simulink model "SYSTEM"  (R2026a)
settings: Solver=VariableStepAuto
model workspace (MAT data in the model file):
  CompAir_P : Simulink.ConnectionBus (value not decoded)
  CompAir_S : Simulink.Bus (value not decoded)
  Control_P : Simulink.ConnectionBus (value not decoded)
  Control_S : Simulink.Bus (value not decoded)
  CoolingFW_P : Simulink.ConnectionBus (value not decoded)
  CoolingFW_S : Simulink.Bus (value not decoded)
  FuelOil_P : Simulink.ConnectionBus (value not decoded)
  FuelOil_S : Simulink.Bus (value not decoded)
  Heat_P : Simulink.ConnectionBus (value not decoded)
  Heat_S : Simulink.Bus (value not decoded)
  LubeOil_P : Simulink.ConnectionBus (value not decoded)
  LubeOil_S : Simulink.Bus (value not decoded)
  Physical : Simulink.ConnectionBus (value not decoded)
  Power_P : Simulink.ConnectionBus (value not decoded)
  Power_S : Simulink.Bus (value not decoded)
  SaltWater_P : Simulink.ConnectionBus (value not decoded)
  SaltWater_S : Simulink.Bus (value not decoded)
  WasteGas_P : Simulink.ConnectionBus (value not decoded)
  WasteGas_S : Simulink.Bus (value not decoded)
  WasteOil_P : Simulink.ConnectionBus (value not decoded)
  WasteOil_S : Simulink.Bus (value not decoded)
  WasteSolid_P : Simulink.ConnectionBus (value not decoded)
  WasteSolid_S : Simulink.Bus (value not decoded)
  WasteWater_P : Simulink.ConnectionBus (value not decoded)
  WasteWater_S : Simulink.Bus (value not decoded)
undefined symbols (not defined in the file): FUEL
(part 4 of 5)

== system SYSTEM/SHIP/200 (PROPULSION)/21X (PROPULSORS) ==
  42X-21XC : Inport  OutDataTypeStr=Bus: Control_S
  51X-21XLO : Inport  Port=2  OutDataTypeStr=Bus: LubeOil_S
  53X-21XCA : Inport  Port=3  OutDataTypeStr=Bus: CompAir_S
  50X-21XCFW : Inport  Port=4  OutDataTypeStr=Bus: CoolingFW_S
  21X ABSENT : Subsystem  VariantControl=21X ABSENT
      settings: PortSchema="{\"entries\":[{\"content\":{\"headerSize\":26,\"margin\":15,\"minimumSpacing\":25,\"sides\":[{\"content\":{},\"type\":\"ConnectorPlacement.EquallySpacedRectSide\",\"uuid\":\"c62bca68-e99b-4d4a-8c3b-c9a3c6520291\"},{\"content\":{\"side\":\"RIGHT\"},\"type\":\"ConnectorPlacement.EquallySpacedRectSide\",\"uuid\":\"9f78cd75-5645-4950-8d66-9f0d33627f1f\"},{\"content\":{\"side\":\"TOP\"},\"type\":\"ConnectorPlacement.EquallySpacedRectSide\",\"uuid\":\"f95077c9-4a6b-4bf1-8b13-59697d659817\"},{\"content\":{\"side\":\"BOTTOM\"},\"type\":\"ConnectorPlacement.EquallySpacedRectSide\",\"uuid\":\"6b5f2b68-9ed2-4485-9686-f8a23585a666\"}]},\"type\":\"ConnectorPlacement.EquallySpacedConnector\",\"uuid\":\"da1ef182-4ed3-4fb4-823f-e8eb0a5ecd15\"}],\"packageUris\":[\"http://schema.mathworks.com/mf0/Connector/R2020b\"],\"version\":\"1.0\"}"
  21X ELECTRIC DRIVE : Subsystem  VariantControl=21X ELECTRIC DRIVE
      settings: PortSchema="{\"entries\":[{\"content\":{\"headerSize\":26,\"margin\":15,\"minimumSpacing\":25,\"sides\":[{\"content\":{\"connectorIds\":[\"Out1\"]},\"type\":\"ConnectorPlacement.EquallySpacedRectSide\",\"uuid\":\"c62bca68-e99b-4d4a-8c3b-c9a3c6520291\"},{\"content\":{\"connectorIds\":[\"In1\"],\"side\":\"RIGHT\"},\"type\":\"ConnectorPlacement.EquallySpacedRectSide\",\"uuid\":\"9f78cd75-5645-4950-8d66-9f0d33627f1f\"},{\"content\":{\"connectorIds\":[\"Out4\",\"Out2\",\"Out3\",\"In4\",\"In2\",\"In3\"],\"side\":\"TOP\"},\"type\":\"ConnectorPlacement.EquallySpacedRectSide\",\"uuid\":\"f95077c9-4a6b-4bf1-8b13-59697d659817\"},{\"content\":{\"connectorIds\":[\"RConn1\",\"RConn2\"],\"side\":\"BOTTOM\"},\"type\":\"ConnectorPlacement.EquallySpacedRectSide\",\"uuid\":\"6b5f2b68-9ed2-4485-9686-f8a23585a666\"}]},\"type\":\"ConnectorPlacement.EquallySpacedConnector\",\"uuid\":\"da1ef182-4ed3-4fb4-823f-e8eb0a5ecd15\"}],\"packageUris\":[\"http://schema.mathworks.com/mf0/Connector/R2020b\"],\"version\":\"1.0\"}"
  21X ELECTRIC DRIVE + MANEUVERING THRUSTER : Subsystem  VariantControl=21X ELECTRIC DRIVE + MANUVERING THRUSTER
      settings: PortSchema="{\"entries\":[{\"content\":{\"headerSize\":26,\"margin\":15,\"minimumSpacing\":25,\"sides\":[{\"content\":{\"connectorIds\":[\"Out1\"]},\"type\":\"ConnectorPlacement.EquallySpacedRectSide\",\"uuid\":\"c62bca68-e99b-4d4a-8c3b-c9a3c6520291\"},{\"content\":{\"connectorIds\":[\"In1\"],\"side\":\"RIGHT\"},\"type\":\"ConnectorPlacement.EquallySpacedRectSide\",\"uuid\":\"9f78cd75-5645-4950-8d66-9f0d33627f1f\"},{\"content\":{\"connectorIds\":[\"Out4\",\"Out2\",\"Out3\",\"In4\",\"In2\",\"In3\"],\"side\":\"TOP\"},\"type\":\"ConnectorPlacement.EquallySpacedRectSide\",\"uuid\":\"f95077c9-4a6b-4bf1-8b13-59697d659817\"},{\"content\":{\"connectorIds\":[\"RConn1\",\"RConn2\"],\"side\":\"BOTTOM\"},\"type\":\"ConnectorPlacement.EquallySpacedRectSide\",\"uuid\":\"6b5f2b68-9ed2-4485-9686-f8a23585a666\"}]},\"type\":\"ConnectorPlacement.EquallySpacedConnector\",\"uuid\":\"da1ef182-4ed3-4fb4-823f-e8eb0a5ecd15\"}],\"packageUris\":[\"http://schema.mathworks.com/mf0/Connector/R2020b\"],\"version\":\"1.0\"}"
  21X SHAFT DRIVE : Subsystem  VariantControl=21X SHAFT DRIVE
      settings: PortSchema="{\"entries\":[{\"content\":{\"headerSize\":26,\"margin\":15,\"minimumSpacing\":25,\"sides\":[{\"content\":{\"connectorIds\":[\"Out1\"]},\"type\":\"ConnectorPlacement.EquallySpacedRectSide\",\"uuid\":\"c62bca68-e99b-4d4a-8c3b-c9a3c6520291\"},{\"content\":{\"connectorIds\":[\"In1\"],\"side\":\"RIGHT\"},\"type\":\"ConnectorPlacement.EquallySpacedRectSide\",\"uuid\":\"9f78cd75-5645-4950-8d66-9f0d33627f1f\"},{\"content\":{\"connectorIds\":[\"Out4\",\"Out2\",\"Out3\",\"In4\",\"In2\",\"In3\"],\"side\":\"TOP\"},\"type\":\"ConnectorPlacement.EquallySpacedRectSide\",\"uuid\":\"f95077c9-4a6b-4bf1-8b13-59697d659817\"},{\"content\":{\"connectorIds\":[\"RConn1\",\"RConn2\"],\"side\":\"BOTTOM\"},\"type\":\"ConnectorPlacement.EquallySpacedRectSide\",\"uuid\":\"6b5f2b68-9ed2-4485-9686-f8a23585a666\"}]},\"type\":\"ConnectorPlacement.EquallySpacedConnector\",\"uuid\":\"da1ef182-4ed3-4fb4-823f-e8eb0a5ecd15\"}],\"packageUris\":[\"http://schema.mathworks.com/mf0/Connector/R2020b\"],\"version\":\"1.0\"}"
  21X SHAFT DRIVE + MANEUVERING THRUSTER : Subsystem  VariantControl=21X SHAFT DRIVE + MANUVERING THRUSTER
      settings: PortSchema="{\"entries\":[{\"content\":{\"headerSize\":26,\"margin\":15,\"minimumSpacing\":25,\"sides\":[{\"content\":{\"connectorIds\":[\"Out1\"]},\"type\":\"ConnectorPlacement.EquallySpacedRectSide\",\"uuid\":\"c62bca68-e99b-4d4a-8c3b-c9a3c6520291\"},{\"content\":{\"connectorIds\":[\"In1\"],\"side\":\"RIGHT\"},\"type\":\"ConnectorPlacement.EquallySpacedRectSide\",\"uuid\":\"9f78cd75-5645-4950-8d66-9f0d33627f1f\"},{\"content\":{\"connectorIds\":[\"Out4\",\"Out2\",\"Out3\",\"In4\",\"In2\",\"In3\"],\"side\":\"TOP\"},\"type\":\"ConnectorPlacement.EquallySpacedRectSide\",\"uuid\":\"f95077c9-4a6b-4bf1-8b13-59697d659817\"},{\"content\":{\"connectorIds\":[\"RConn1\",\"RConn2\"],\"side\":\"BOTTOM\"},\"type\":\"ConnectorPlacement.EquallySpacedRectSide\",\"uuid\":\"6b5f2b68-9ed2-4485-9686-f8a23585a666\"}]},\"type\":\"ConnectorPlacement.EquallySpacedConnector\",\"uuid\":\"da1ef182-4ed3-4fb4-823f-e8eb0a5ecd15\"}],\"packageUris\":[\"http://schema.mathworks.com/mf0/Connector/R2020b\"],\"version\":\"1.0\"}"
  21X WATER JET : Subsystem  VariantControl=21X WATER JET
      settings: PortSchema="{\"entries\":[{\"content\":{\"headerSize\":26,\"margin\":15,\"minimumSpacing\":25,\"sides\":[{\"content\":{\"connectorIds\":[\"Out1\"]},\"type\":\"ConnectorPlacement.EquallySpacedRectSide\",\"uuid\":\"c62bca68-e99b-4d4a-8c3b-c9a3c6520291\"},{\"content\":{\"connectorIds\":[\"In1\"],\"side\":\"RIGHT\"},\"type\":\"ConnectorPlacement.EquallySpacedRectSide\",\"uuid\":\"9f78cd75-5645-4950-8d66-9f0d33627f1f\"},{\"content\":{\"connectorIds\":[\"Out4\",\"Out2\",\"Out3\",\"In4\",\"In2\",\"In3\"],\"side\":\"TOP\"},\"type\":\"ConnectorPlacement.EquallySpacedRectSide\",\"uuid\":\"f95077c9-4a6b-4bf1-8b13-59697d659817\"},{\"content\":{\"connectorIds\":[\"RConn1\",\"RConn2\"],\"side\":\"BOTTOM\"},\"type\":\"ConnectorPlacement.EquallySpacedRectSide\",\"uuid\":\"6b5f2b68-9ed2-4485-9686-f8a23585a666\"}]},\"type\":\"ConnectorPlacement.EquallySpacedConnector\",\"uuid\":\"da1ef182-4ed3-4fb4-823f-e8eb0a5ecd15\"}],\"packageUris\":[\"http://schema.mathworks.com/mf0/Connector/R2020b\"],\"version\":\"1.0\"}"
  21X WATER JET + MANEUVERING THRUSTER : Subsystem  VariantControl=21X WATER JET + MANUVERING THRUSTER
      settings: PortSchema="{\"entries\":[{\"content\":{\"headerSize\":26,\"margin\":15,\"minimumSpacing\":25,\"sides\":[{\"content\":{\"connectorIds\":[\"Out1\"]},\"type\":\"ConnectorPlacement.EquallySpacedRectSide\",\"uuid\":\"c62bca68-e99b-4d4a-8c3b-c9a3c6520291\"},{\"content\":{\"connectorIds\":[\"In1\"],\"side\":\"RIGHT\"},\"type\":\"ConnectorPlacement.EquallySpacedRectSide\",\"uuid\":\"9f78cd75-5645-4950-8d66-9f0d33627f1f\"},{\"content\":{\"connectorIds\":[\"Out4\",\"Out2\",\"Out3\",\"In4\",\"In2\",\"In3\"],\"side\":\"TOP\"},\"type\":\"ConnectorPlacement.EquallySpacedRectSide\",\"uuid\":\"f95077c9-4a6b-4bf1-8b13-59697d659817\"},{\"content\":{\"connectorIds\":[\"RConn1\",\"RConn2\"],\"side\":\"BOTTOM\"},\"type\":\"ConnectorPlacement.EquallySpacedRectSide\",\"uuid\":\"6b5f2b68-9ed2-4485-9686-f8a23585a666\"}]},\"type\":\"ConnectorPlacement.EquallySpacedConnector\",\"uuid\":\"da1ef182-4ed3-4fb4-823f-e8eb0a5ecd15\"}],\"packageUris\":[\"http://schema.mathworks.com/mf0/Connector/R2020b\"],\"version\":\"1.0\"}"
  10X-21X : PMIOPort  Side=Right  ConnectionType=Bus: Physical
  FROM 22X : PMIOPort  Port=2  Side=Right  ConnectionType=Bus: Physical
  21X-42XC : Outport  OutDataTypeStr=Bus: Control_S
  21X-51XLO : Outport  Port=2  OutDataTypeStr=Bus: LubeOil_S
  21X-53XCA : Outport  Port=3  OutDataTypeStr=Bus: CompAir_S
  21X-50XCFW : Outport  Port=4  OutDataTypeStr=Bus: CoolingFW_S

== system SYSTEM/SHIP/200 (PROPULSION)/22X (SHAFTING) ==
  51X-22XLO : Inport  OutDataTypeStr=Bus: LubeOil_S
  53X-22XCA : Inport  Port=2  OutDataTypeStr=Bus: CompAir_S
  22X ABSENT : Subsystem  VariantControl=22X ABSENT
      settings: PortSchema="{\"entries\":[{\"content\":{\"headerSize\":26,\"margin\":15,\"minimumSpacing\":25,\"sides\":[{\"content\":{},\"type\":\"ConnectorPlacement.EquallySpacedRectSide\",\"uuid\":\"c62bca68-e99b-4d4a-8c3b-c9a3c6520291\"},{\"content\":{\"side\":\"RIGHT\"},\"type\":\"ConnectorPlacement.EquallySpacedRectSide\",\"uuid\":\"9f78cd75-5645-4950-8d66-9f0d33627f1f\"},{\"content\":{\"side\":\"TOP\"},\"type\":\"ConnectorPlacement.EquallySpacedRectSide\",\"uuid\":\"f95077c9-4a6b-4bf1-8b13-59697d659817\"},{\"content\":{\"side\":\"BOTTOM\"},\"type\":\"ConnectorPlacement.EquallySpacedRectSide\",\"uuid\":\"1f93f758-4269-498d-aa3c-a1654d57bbcc\"}]},\"type\":\"ConnectorPlacement.EquallySpacedConnector\",\"uuid\":\"da1ef182-4ed3-4fb4-823f-e8eb0a5ecd15\"}],\"packageUris\":[\"http://schema.mathworks.com/mf0/Connector/R2020b\"],\"version\":\"1.0\"}"
  22X MECHANICAL : Subsystem  VariantControl=22X MECHANICAL
      settings: PortSchema="{\"entries\":[{\"content\":{\"headerSize\":26,\"margin\":15,\"minimumSpacing\":25,\"sides\":[{\"content\":{\"connectorIds\":[\"Out3\"]},\"type\":\"ConnectorPlacement.EquallySpacedRectSide\",\"uuid\":\"c62bca68-e99b-4d4a-8c3b-c9a3c6520291\"},{\"content\":{\"side\":\"RIGHT\"},\"type\":\"ConnectorPlacement.EquallySpacedRectSide\",\"uuid\":\"9f78cd75-5645-4950-8d66-9f0d33627f1f\"},{\"content\":{\"connectorIds\":[\"Out1\",\"Out2\",\"In1\",\"In2\"],\"side\":\"TOP\"},\"type\":\"ConnectorPlacement.EquallySpacedRectSide\",\"uuid\":\"f95077c9-4a6b-4bf1-8b13-59697d659817\"},{\"content\":{\"connectorIds\":[\"RConn3\",\"RConn2\",\"RConn1\"],\"side\":\"BOTTOM\"},\"type\":\"ConnectorPlacement.EquallySpacedRectSide\",\"uuid\":\"1f93f758-4269-498d-aa3c-a1654d57bbcc\"}]},\"type\":\"ConnectorPlacement.EquallySpacedConnector\",\"uuid\":\"da1ef182-4ed3-4fb4-823f-e8eb0a5ecd15\"}],\"packageUris\":[\"http://schema.mathworks.com/mf0/Connector/R2020b\"],\"version\":\"1.0\"}"
  TOFROM 23X : PMIOPort  Side=Right  ConnectionType=Bus: Physical
  10X-22X : PMIOPort  Port=2  Side=Right  ConnectionType=Bus: Physical
  TO 21X : PMIOPort  Port=3  Side=Right  ConnectionType=Bus: Physical
  22X-51XLO : Outport  OutDataTypeStr=Bus: LubeOil_S
  22X-53XCA : Outport  Port=2  OutDataTypeStr=Bus: CompAir_S
  22X-42XC : Outport  Port=3  OutDataTypeStr=Bus: Control_S

== system SYSTEM/SHIP/200 (PROPULSION)/23X (POWER TRANSMISSION) ==
  51X-23XLO : Inport  OutDataTypeStr=Bus: LubeOil_S
  42X-23XC : Inport  Port=2  OutDataTypeStr=Bus: Control_S
  23X ABSENT : Subsystem  VariantControl=23X ABSENT
      settings: PortSchema="{\"entries\":[{\"content\":{\"headerSize\":26,\"margin\":15,\"minimumSpacing\":25,\"sides\":[{\"content\":{},\"type\":\"ConnectorPlacement.EquallySpacedRectSide\",\"uuid\":\"c62bca68-e99b-4d4a-8c3b-c9a3c6520291\"},{\"content\":{\"side\":\"RIGHT\"},\"type\":\"ConnectorPlacement.EquallySpacedRectSide\",\"uuid\":\"9f78cd75-5645-4950-8d66-9f0d33627f1f\"},{\"content\":{\"side\":\"TOP\"},\"type\":\"ConnectorPlacement.EquallySpacedRectSide\",\"uuid\":\"f95077c9-4a6b-4bf1-8b13-59697d659817\"},{\"content\":{\"side\":\"BOTTOM\"},\"type\":\"ConnectorPlacement.EquallySpacedRectSide\",\"uuid\":\"886e986c-d088-4ccd-a11a-30cba32770e8\"}]},\"type\":\"ConnectorPlacement.EquallySpacedConnector\",\"uuid\":\"da1ef182-4ed3-4fb4-823f-e8eb0a5ecd15\"}],\"packageUris\":[\"http://schema.mathworks.com/mf0/Connector/R2020b\"],\"version\":\"1.0\"}"
  23X MECHANICAL : Subsystem  VariantControl=23X MECHANICAL
      settings: PortSchema="{\"entries\":[{\"content\":{\"headerSize\":26,\"margin\":15,\"minimumSpacing\":25,\"sides\":[{\"content\":{\"connectorIds\":[\"Out2\"]},\"type\":\"ConnectorPlacement.EquallySpacedRectSide\",\"uuid\":\"c62bca68-e99b-4d4a-8c3b-c9a3c6520291\"},{\"content\":{\"connectorIds\":[\"Out3\",\"In2\"],\"side\":\"RIGHT\"},\"type\":\"ConnectorPlacement.EquallySpacedRectSide\",\"uuid\":\"9f78cd75-5645-4950-8d66-9f0d33627f1f\"},{\"content\":{\"connectorIds\":[\"Out1\",\"In1\"],\"side\":\"TOP\"},\"type\":\"ConnectorPlacement.EquallySpacedRectSide\",\"uuid\":\"f95077c9-4a6b-4bf1-8b13-59697d659817\"},{\"content\":{\"connectorIds\":[\"LConn2\",\"LConn1\",\"RConn1\"],\"side\":\"BOTTOM\"},\"type\":\"ConnectorPlacement.EquallySpacedRectSide\",\"uuid\":\"886e986c-d088-4ccd-a11a-30cba32770e8\"}]},\"type\":\"ConnectorPlacement.EquallySpacedConnector\",\"uuid\":\"da1ef182-4ed3-4fb4-823f-e8eb0a5ecd15\"}],\"packageUris\":[\"http://schema.mathworks.com/mf0/Connector/R2020b\"],\"version\":\"1.0\"}"
  23X MECHANICAL WITH POWER TAKEOFF : Subsystem  VariantControl=23X MECHANICAL WITH POWER TAKEOFF
      settings: PortSchema="{\"entries\":[{\"content\":{\"headerSize\":26,\"margin\":15,\"minimumSpacing\":25,\"sides\":[{\"content\":{\"connectorIds\":[\"Out2\"]},\"type\":\"ConnectorPlacement.EquallySpacedRectSide\",\"uuid\":\"c62bca68-e99b-4d4a-8c3b-c9a3c6520291\"},{\"content\":{\"connectorIds\":[\"Out3\",\"In2\"],\"side\":\"RIGHT\"},\"type\":\"ConnectorPlacement.EquallySpacedRectSide\",\"uuid\":\"9f78cd75-5645-4950-8d66-9f0d33627f1f\"},{\"content\":{\"connectorIds\":[\"Out1\",\"In1\"],\"side\":\"TOP\"},\"type\":\"ConnectorPlacement.EquallySpacedRectSide\",\"uuid\":\"f95077c9-4a6b-4bf1-8b13-59697d659817\"},{\"content\":{\"connectorIds\":[\"LConn2\",\"LConn1\",\"RConn1\"],\"side\":\"BOTTOM\"},\"type\":\"ConnectorPlacement.EquallySpacedRectSide\",\"uuid\":\"886e986c-d088-4ccd-a11a-30cba32770e8\"}]},\"type\":\"ConnectorPlacement.EquallySpacedConnector\",\"uuid\":\"da1ef182-4ed3-4fb4-823f-e8eb0a5ecd15\"}],\"packageUris\":[\"http://schema.mathworks.com/mf0/Connector/R2020b\"],\"version\":\"1.0\"}"
  TOFROM 22X : PMIOPort  Side=Left  ConnectionType=Bus: Physical
  FROM 20X : PMIOPort  Port=2  Side=Left  ConnectionType=Bus: Physical
  10X-23X : PMIOPort  Port=3  Side=Right  ConnectionType=Bus: Physical
  23X-51XLO : Outport  OutDataTypeStr=Bus: LubeOil_S
  23X-42XC : Outport  Port=2  OutDataTypeStr=Bus: Control_S
  23X-31XP : Outport  Port=3  OutDataTypeStr=Bus: Power_S

== system SYSTEM/SHIP/300 (ELECTRICAL)/30X (GENERATOR SETS) ==
  Bus Element In1 : Inport  PortName=42X-30XC
  Bus Element In3 : Inport  Port=2  PortName=51X-30XLO
  Bus Element In5 : Inport  Port=3  PortName=53X-30XCA
  Bus Element In4 : Inport  Port=4  PortName=52X-30XFO
  Bus Element In2 : Inport  Port=5  PortName=50X-30XCFW
  10X-30X : PMIOPort  Side=Right  ConnectionType=Bus: Physical
  30X-526FO : PMIOPort  Port=2  Side=Left  ConnectionType=Bus: FuelOil_P
  526-30XFO : PMIOPort  Port=3  Side=Left  ConnectionType=Bus: FuelOil_P
  Bus Element Out2 : Outport  PortName=30X-42XC
  Bus Element Out4 : Outport  Port=2  PortName=30X-51XLO
  Bus Element Out5 : Outport  Port=3  PortName=30X-52XFO
  Bus Element Out6 : Outport  Port=4  PortName=30X-53XCA
  Bus Element Out7 : Outport  Port=5  PortName=30X-57XWG
  Bus Element Out3 : Outport  Port=6  PortName=30X-50XCFW
  Bus Element Out1 : Outport  Port=7  PortName=30X-31XP

== system SYSTEM/SHIP/300 (ELECTRICAL)/31X (POWER DISTRIBUTION) ==
  Bus Element In3 : Inport  PortName=23X-31XP
  Bus Element In4 : Inport  Port=2  PortName=32X-31XP
  Bus Element In5 : Inport  Port=3  PortName=42X-31XC
  Bus Element In1 : Inport  Port=4  PortName=30X-31XP
  Bus Element In2 : Inport  Port=5  PortName=33X-31XP
  10X-31X : PMIOPort  Side=Right  ConnectionType=Bus: Physical
  Bus Element Out25 : Outport  PortName=31X-42XC
  Bus Element Out3 : Outport  Port=2  PortName=31X-40XP
  Bus Element Out4 : Outport  Port=3  PortName=31X-41XP
  Bus Element Out5 : Outport  Port=4  PortName=31X-42XP
  Bus Element Out6 : Outport  Port=5  PortName=31X-43XP
  Bus Element Out7 : Outport  Port=6  PortName=31X-44XP
  Bus Element Out2 : Outport  Port=7  PortName=31X-45XP
  Bus Element Out8 : Outport  Port=8  PortName=31X-50XP
  Bus Element Out9 : Outport  Port=9  PortName=31X-51XP
  Bus Element Out10 : Outport  Port=10  PortName=31X-529P
  Bus Element Out11 : Outport  Port=11  PortName=31X-53XP
  Bus Element Out12 : Outport  Port=12  PortName=31X-54XP
  Bus Element Out13 : Outport  Port=13  PortName=31X-55XP
  Bus Element Out14 : Outport  Port=14  PortName=31X-56XP
  Bus Element Out15 : Outport  Port=15  PortName=31X-57XP
  Bus Element Out16 : Outport  Port=16  PortName=31X-58XP
  Bus Element Out17 : Outport  Port=17  PortName=31X-59XP
  Bus Element Out18 : Outport  Port=18  PortName=31X-60XP
  Bus Element Out19 : Outport  Port=19  PortName=31X-61XP
  Bus Element Out20 : Outport  Port=20  PortName=31X-70XP
  Bus Element Out21 : Outport  Port=21  PortName=31X-71XP
  Bus Element Out22 : Outport  Port=22  PortName=31X-72XP
  Bus Element Out23 : Outport  Port=23  PortName=31X-73XP
  Bus Element Out24 : Outport  Port=24  PortName=31X-74XP
  Bus Element Out1 : Outport  Port=25  PortName=31X-32XP

== system SYSTEM/SHIP/300 (ELECTRICAL)/32X (BATTERY) ==
  Bus Element In2 : Inport  PortName=42X-32XC
  Bus Element In1 : Inport  Port=2  PortName=31X-32XP
  10X-32X : PMIOPort  Side=Right  ConnectionType=Bus: Physical
  Bus Element Out1 : Outport  PortName=32X-31XP
  Bus Element Out2 : Outport  Port=2  PortName=32X-42XC

== system SYSTEM/SHIP/300 (ELECTRICAL)/33X (SHORE POWER) ==
  Bus Element In1 : Inport  PortName=42X-33XC
  10X-33X : PMIOPort  Side=Right  ConnectionType=Bus: Physical
  Bus Element Out2 : Outport  PortName=33X-42XC
  Bus Element Out1 : Outport  Port=2  PortName=33X-31XP

== system SYSTEM/SHIP/400 (COMMAND CONTROL)/40X (NAVIGATION//AIS) ==
  Bus Element In3 : Inport  PortName=53X-40XCA
  Bus Element In2 : Inport  Port=2  PortName=42X-40XC
  Bus Element In1 : Inport  Port=3  PortName=31X-40XP
  10X-40X : PMIOPort  Side=Right  ConnectionType=Bus: Physical
  Bus Element Out2 : Outport  PortName=40X-53XCA
  Bus Element Out1 : Outport  Port=2  PortName=40X-42XC

== system SYSTEM/SHIP/400 (COMMAND CONTROL)/41X (RADIO//SATCOM) ==
  Bus Element In2 : Inport  PortName=42X-41XC
  Bus Element In1 : Inport  Port=2  PortName=31X-41XP
  10X-41X : PMIOPort  Side=Right  ConnectionType=Bus: Physical
  Bus Element Out1 : Outport  PortName=41X-42XC

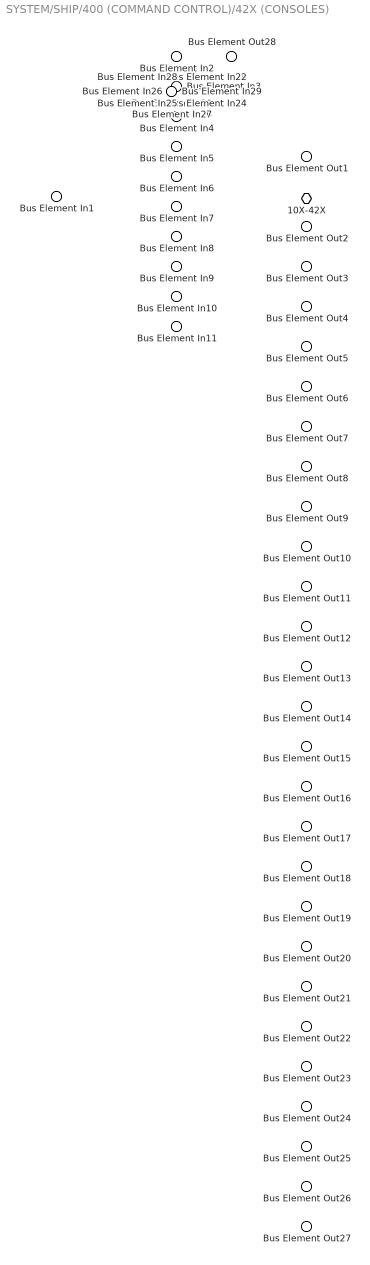
== system SYSTEM/SHIP/400 (COMMAND CONTROL)/42X (CONSOLES) ==
  Bus Element In30 : Inport  PortName=50X-42XCFW
  Bus Element In2 : Inport  Port=2  PortName=41X-42XC
  Bus Element In3 : Inport  Port=3  PortName=40X-42XC
  Bus Element In4 : Inport  Port=4  PortName=43X-42XC
  Bus Element In5 : Inport  Port=5  PortName=44X-42XC
  Bus Element In6 : Inport  Port=6  PortName=45X-42XC
  Bus Element In7 : Inport  Port=7  PortName=20X-42XC
  Bus Element In8 : Inport  Port=8  PortName=21X-42XC
  Bus Element In10 : Inport  Port=9  PortName=22X-42XC
  Bus Element In9 : Inport  Port=10  PortName=23X-42XC
  Bus Element In11 : Inport  Port=11  PortName=30X-42XC
  Bus Element In12 : Inport  Port=12  PortName=31X-42XC
  Bus Element In13 : Inport  Port=13  PortName=32X-42XC
  Bus Element In14 : Inport  Port=14  PortName=33X-42XC
  Bus Element In15 : Inport  Port=15  PortName=50X-42XC
  Bus Element In16 : Inport  Port=16  PortName=51X-42XC
  Bus Element In17 : Inport  Port=17  PortName=528-42XC
  Bus Element In18 : Inport  Port=18  PortName=53X-42XC
  Bus Element In19 : Inport  Port=19  PortName=54X-42XC
  Bus Element In20 : Inport  Port=20  PortName=55X-42XC
  Bus Element In21 : Inport  Port=21  PortName=56X-42XC
  Bus Element In22 : Inport  Port=22  PortName=57X-42XC
  Bus Element In23 : Inport  Port=23  PortName=58X-42XC
  Bus Element In24 : Inport  Port=24  PortName=59X-42XC
  Bus Element In25 : Inport  Port=25  PortName=70X-42XC
  Bus Element In26 : Inport  Port=26  PortName=71X-42XC
  Bus Element In27 : Inport  Port=27  PortName=72X-42XC
  Bus Element In28 : Inport  Port=28  PortName=73X-42XC
  Bus Element In29 : Inport  Port=29  PortName=74X-42XC
  Bus Element In1 : Inport  Port=30  PortName=31X-42XP
  10X-42X : PMIOPort  Side=Right  ConnectionType=Bus: Physical
  Bus Element Out28 : Outport  PortName=42X-50XCFW
  Bus Element Out1 : Outport  Port=2  PortName=42X-40XC
  Bus Element Out2 : Outport  Port=3  PortName=42X-41XC
  Bus Element Out3 : Outport  Port=4  PortName=42X-43XC
  Bus Element Out4 : Outport  Port=5  PortName=42X-44XC
  Bus Element Out5 : Outport  Port=6  PortName=42X-45XC
  Bus Element Out6 : Outport  Port=7  PortName=42X-20XC
  Bus Element Out7 : Outport  Port=8  PortName=42X-21XC
  Bus Element Out8 : Outport  Port=9  PortName=42X-23XC
  Bus Element Out9 : Outport  Port=10  PortName=42X-30XC
  Bus Element Out10 : Outport  Port=11  PortName=42X-31XC
  Bus Element Out11 : Outport  Port=12  PortName=42X-32XC
  Bus Element Out12 : Outport  Port=13  PortName=42X-33XC
  Bus Element Out13 : Outport  Port=14  PortName=42X-50XC
  Bus Element Out14 : Outport  Port=15  PortName=42X-51XC
  Bus Element Out15 : Outport  Port=16  PortName=42X-528C
  Bus Element Out16 : Outport  Port=17  PortName=42X-53XC
  Bus Element Out17 : Outport  Port=18  PortName=42X-54XC
  Bus Element Out18 : Outport  Port=19  PortName=42X-55XC
  Bus Element Out19 : Outport  Port=20  PortName=42X-56XC
  Bus Element Out20 : Outport  Port=21  PortName=42X-57XC
  Bus Element Out21 : Outport  Port=22  PortName=42X-58XC
  Bus Element Out22 : Outport  Port=23  PortName=42X-59XC
  Bus Element Out23 : Outport  Port=24  PortName=42X-70XC
  Bus Element Out24 : Outport  Port=25  PortName=42X-71XC
  Bus Element Out25 : Outport  Port=26  PortName=42X-72XC
  Bus Element Out26 : Outport  Port=27  PortName=42X-73XC
  Bus Element Out27 : Outport  Port=28  PortName=42X-74XC

== system SYSTEM/SHIP/400 (COMMAND CONTROL)/43X (STEERAGE) ==
  Bus Element In2 : Inport  PortName=42X-43XC
  Bus Element In4 : Inport  Port=2  PortName=51X-43XLO
  Bus Element In3 : Inport  Port=3  PortName=50X-43XCFW
  Bus Element In1 : Inport  Port=4  PortName=31X-43XP
  10X-43X : PMIOPort  Side=Right  ConnectionType=Bus: Physical
  Bus Element Out1 : Outport  PortName=43X-42XC
  Bus Element Out3 : Outport  Port=2  PortName=43X-51XLO
  Bus Element Out2 : Outport  Port=3  PortName=43X-50XCFW

== system SYSTEM/SHIP/400 (COMMAND CONTROL)/44X (AIR SURVEILLANCE) ==
  Bus Element In3 : Inport  PortName=50X-44XCFW
  Bus Element In2 : Inport  Port=2  PortName=42X-44XC
  Bus Element In1 : Inport  Port=3  PortName=31X-44XP
  10X-44X : PMIOPort  Side=Right  ConnectionType=Bus: Physical
  Bus Element Out2 : Outport  PortName=44X-50XCFW
  Bus Element Out1 : Outport  Port=2  PortName=44X-42XC

== system SYSTEM/SHIP/400 (COMMAND CONTROL)/45X (WATER SURVEILLANCE) ==
  Bus Element In2 : Inport  PortName=42X-45XC
  Bus Element In1 : Inport  Port=2  PortName=31X-45XP
  10X-45X : PMIOPort  Side=Right  ConnectionType=Bus: Physical
  Bus Element Out1 : Outport  PortName=45X-42XC

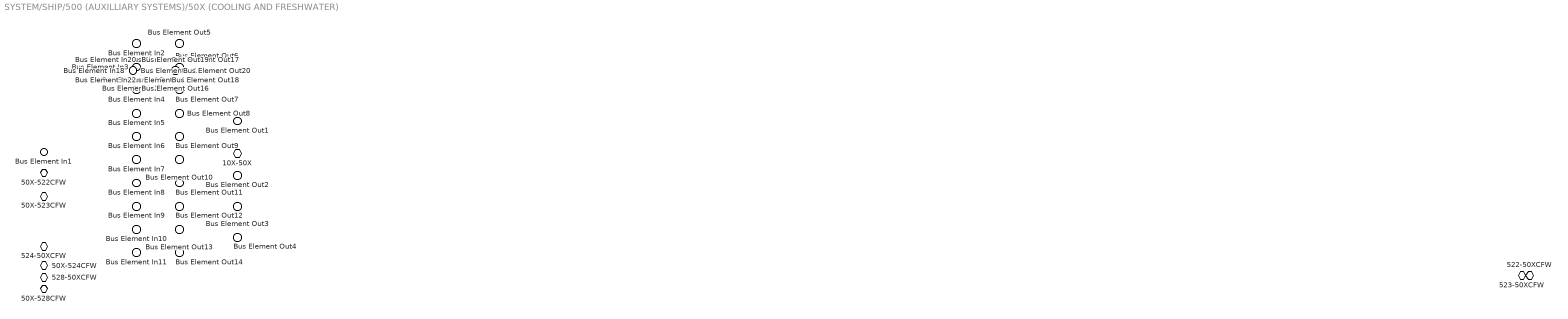
== system SYSTEM/SHIP/500 (AUXILLIARY SYSTEMS)/50X (COOLING AND FRESHWATER) ==
  Bus Element In2 : Inport  PortName=42X-50XC
  Bus Element In3 : Inport  Port=2  PortName=20X-50XCFW
  Bus Element In4 : Inport  Port=3  PortName=21X-50XCFW
  Bus Element In16 : Inport  Port=4  PortName=42X-50XCFW
  Bus Element In6 : Inport  Port=5  PortName=43X-50XCFW
  Bus Element In17 : Inport  Port=6  PortName=44X-50XCFW
  Bus Element In7 : Inport  Port=7  PortName=51X-50XCFW
  Bus Element In23 : Inport  Port=8  PortName=51X-50XLO
  Bus Element In8 : Inport  Port=9  PortName=52X-50XCFW
  Bus Element In9 : Inport  Port=10  PortName=53X-50XCFW
  Bus Element In10 : Inport  Port=11  PortName=54X-50XSW
  Bus Element In11 : Inport  Port=12  PortName=54X-50XCFW
  Bus Element In12 : Inport  Port=13  PortName=55X-50XCFW
  Bus Element In13 : Inport  Port=14  PortName=57X-50XCFW
  Bus Element In14 : Inport  Port=15  PortName=58X-50XCFW
  Bus Element In15 : Inport  Port=16  PortName=59X-50XCFW
  Bus Element In22 : Inport  Port=17  PortName=60X-50XCFW
  Bus Element In21 : Inport  Port=18  PortName=61X-50XCFW
  Bus Element In20 : Inport  Port=19  PortName=71X-50XCFW
  Bus Element In19 : Inport  Port=20  PortName=72X-50XCFW
  Bus Element In18 : Inport  Port=21  PortName=73X-50XCFW
  Bus Element In5 : Inport  Port=22  PortName=30X-50XCFW
  Bus Element In1 : Inport  Port=23  PortName=31X-50XP
  10X-50X : PMIOPort  Side=Right  ConnectionType=Bus: Physical
  50X-522CFW : PMIOPort  Port=2  Side=Left  ConnectionType=Bus: CoolingFW_P
  50X-523CFW : PMIOPort  Port=3  Side=Left  ConnectionType=Bus: CoolingFW_P
  50X-524CFW : PMIOPort  Port=4  Side=Left  ConnectionType=Bus: CoolingFW_P
  50X-528CFW : PMIOPort  Port=5  Side=Left  ConnectionType=Bus: CoolingFW_P
  522-50XCFW : PMIOPort  Port=6  Side=Left  ConnectionType=Bus: CoolingFW_P
  523-50XCFW : PMIOPort  Port=7  Side=Left  ConnectionType=Bus: CoolingFW_P
  524-50XCFW : PMIOPort  Port=8  Side=Left  ConnectionType=Bus: CoolingFW_P
  528-50XCFW : PMIOPort  Port=9  Side=Left  ConnectionType=Bus: CoolingFW_P
  Bus Element Out1 : Outport  PortName=50X-42XC
  Bus Element Out2 : Outport  Port=2  PortName=50X-20XCFW
  Bus Element Out3 : Outport  Port=3  PortName=50X-21XCFW
  Bus Element Out14 : Outport  Port=4  PortName=50X-42XCFW
  Bus Element Out5 : Outport  Port=5  PortName=50X-43XCFW
  Bus Element Out15 : Outport  Port=6  PortName=50X-44XCFW
  Bus Element Out6 : Outport  Port=7  PortName=50X-51XCFW
  Bus Element Out21 : Outport  Port=8  PortName=50X-51XLO
  Bus Element Out7 : Outport  Port=9  PortName=50X-52XCFW
  Bus Element Out8 : Outport  Port=10  PortName=50X-53XCFW
  Bus Element Out9 : Outport  Port=11  PortName=50X-54XCFW
  Bus Element Out10 : Outport  Port=12  PortName=50X-55XCFW
  Bus Element Out11 : Outport  Port=13  PortName=50X-57XCFW
  Bus Element Out12 : Outport  Port=14  PortName=50X-58XCFW
  Bus Element Out13 : Outport  Port=15  PortName=50X-59XCFW
  Bus Element Out16 : Outport  Port=16  PortName=50X-60XCFW
  Bus Element Out17 : Outport  Port=17  PortName=50X-61XCFW
  Bus Element Out18 : Outport  Port=18  PortName=50X-71XCFW
  Bus Element Out19 : Outport  Port=19  PortName=50X-72XCFW
  Bus Element Out20 : Outport  Port=20  PortName=50X-73XCFW
  Bus Element Out4 : Outport  Port=21  PortName=50X-30XCFW

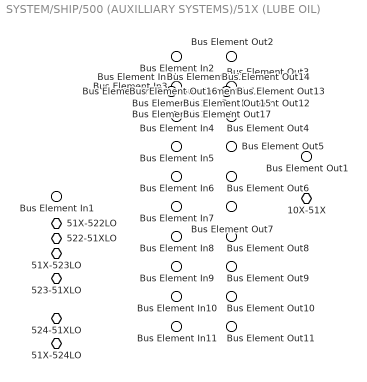
== system SYSTEM/SHIP/500 (AUXILLIARY SYSTEMS)/51X (LUBE OIL) ==
  Bus Element In4 : Inport  PortName=20X-51XLO
  Bus Element In5 : Inport  Port=2  PortName=21X-51XLO
  Bus Element In6 : Inport  Port=3  PortName=22X-51XLO
  Bus Element In7 : Inport  Port=4  PortName=23X-51XLO
  Bus Element In8 : Inport  Port=5  PortName=30X-51XLO
  Bus Element In9 : Inport  Port=6  PortName=43X-51XLO
  Bus Element In3 : Inport  Port=7  PortName=50X-51XCFW
  Bus Element In10 : Inport  Port=8  PortName=50X-51XLO
  Bus Element In11 : Inport  Port=9  PortName=52X-51XLO
  Bus Element In12 : Inport  Port=10  PortName=53X-51XLO
  Bus Element In13 : Inport  Port=11  PortName=54X-51XLO
  Bus Element In14 : Inport  Port=12  PortName=55X-51XLO
  Bus Element In15 : Inport  Port=13  PortName=57X-51XLO
  Bus Element In16 : Inport  Port=14  PortName=58X-51XLO
  Bus Element In17 : Inport  Port=15  PortName=59X-51XLO
  Bus Element In2 : Inport  Port=16  PortName=42X-51XC
  Bus Element In1 : Inport  Port=17  PortName=31X-51XP
  10X-51X : PMIOPort  Side=Right  ConnectionType=Bus: Physical
  51X-522LO : PMIOPort  Port=2  Side=Left  ConnectionType=Bus: LubeOil_P
  51X-523LO : PMIOPort  Port=3  Side=Left  ConnectionType=Bus: LubeOil_P
  51X-524LO : PMIOPort  Port=4  Side=Left  ConnectionType=Bus: LubeOil_P
  522-51XLO : PMIOPort  Port=5  Side=Left  ConnectionType=Bus: LubeOil_P
  523-51XLO : PMIOPort  Port=6  Side=Left  ConnectionType=Bus: LubeOil_P
  524-51XLO : PMIOPort  Port=7  Side=Left  ConnectionType=Bus: LubeOil_P
  Bus Element Out3 : Outport  PortName=51X-20XLO
  Bus Element Out4 : Outport  Port=2  PortName=51X-21XLO
  Bus Element Out5 : Outport  Port=3  PortName=51X-22XLO
  Bus Element Out6 : Outport  Port=4  PortName=51X-23XLO
  Bus Element Out7 : Outport  Port=5  PortName=51X-30XLO
  Bus Element Out8 : Outport  Port=6  PortName=51X-43XLO
  Bus Element Out2 : Outport  Port=7  PortName=51X-50XCFW
  Bus Element Out9 : Outport  Port=8  PortName=51X-50XLO
  Bus Element Out10 : Outport  Port=9  PortName=51X-52XLO
  Bus Element Out11 : Outport  Port=10  PortName=51X-53XLO
  Bus Element Out12 : Outport  Port=11  PortName=51X-54XLO
  Bus Element Out13 : Outport  Port=12  PortName=51X-55XLO
  Bus Element Out17 : Outport  Port=13  PortName=51X-57XWO
  Bus Element Out14 : Outport  Port=14  PortName=51X-57XLO
  Bus Element Out15 : Outport  Port=15  PortName=51X-58XLO
  Bus Element Out16 : Outport  Port=16  PortName=51X-59XLO
  Bus Element Out1 : Outport  Port=17  PortName=51X-42XC

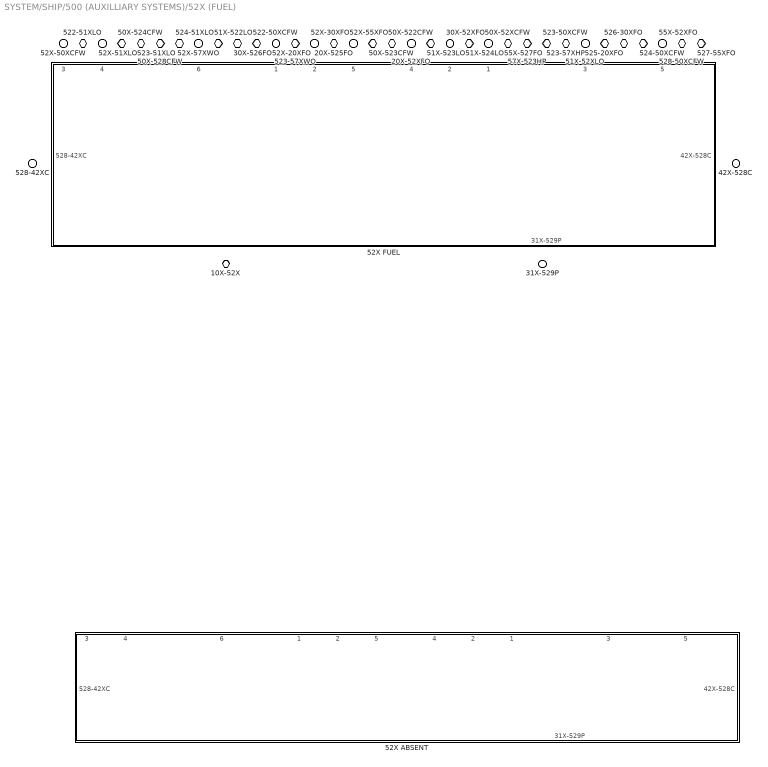
== system SYSTEM/SHIP/500 (AUXILLIARY SYSTEMS)/52X (FUEL) ==
  50X-52XCFW : Inport  OutDataTypeStr=Bus: CoolingFW_S
  30X-52XFO : Inport  Port=2  OutDataTypeStr=Bus: FuelOil_S
  51X-52XLO : Inport  Port=3  OutDataTypeStr=Bus: LubeOil_S
  20X-52XFO : Inport  Port=4  OutDataTypeStr=Bus: FuelOil_S
  55X-52XFO : Inport  Port=5  OutDataTypeStr=Bus: FuelOil_S
  42X-528C : Inport  Port=6  OutDataTypeStr=Bus: Control_S
  31X-529P : Inport  Port=7  OutDataTypeStr=Bus: Power_S
  52X ABSENT : Subsystem  VariantControl=52X ABSENT
      settings: PortSchema="{\"entries\":[{\"content\":{\"headerSize\":26,\"margin\":15,\"minimumSpacing\":25,\"sides\":[{\"content\":{\"connectorIds\":[\"Out7\"]},\"type\":\"ConnectorPlacement.EquallySpacedRectSide\",\"uuid\":\"c62bca68-e99b-4d4a-8c3b-c9a3c6520291\"},{\"content\":{\"connectorIds\":[\"In6\"],\"side\":\"RIGHT\"},\"type\":\"ConnectorPlacement.EquallySpacedRectSide\",\"uuid\":\"9f78cd75-5645-4950-8d66-9f0d33627f1f\"},{\"content\":{\"connectorIds\":[\"Out3\",\"LConn1\",\"Out4\",\"LConn9\",\"LConn2\",\"LConn10\",\"LConn3\",\"Out6\",\"LConn12\",\"LConn6\",\"LConn11\",\"Out1\",\"LConn4\",\"Out2\",\"LConn5\",\"Out5\",\"LConn8\",\"LConn7\",\"In4\",\"LConn13\",\"In2\",\"LConn14\",\"In1\",\"LConn15\",\"LConn16\",\"LConn17\",\"LConn18\",\"In3\",\"LConn19\",\"LConn20\",\"LConn21\",\"In5\",\"LConn22\",\"LConn23\"],\"side\":\"TOP\"},\"type\":\"ConnectorPlacement.EquallySpacedRectSide\",\"uuid\":\"f95077c9-4a6b-4bf1-8b13-59697d659817\"},{\"content\":{\"connectorIds\":[\"RConn1\",\"In7\"],\"side\":\"BOTTOM\"},\"type\":\"ConnectorPlacement.EquallySpacedRectSide\",\"uuid\":\"ebf76d24-9f66-4d93-ad0f-b873a6db50be\"}]},\"type\":\"ConnectorPlacement.EquallySpacedConnector\",\"uuid\":\"da1ef182-4ed3-4fb4-823f-e8eb0a5ecd15\"}],\"packageUris\":[\"http://schema.mathworks.com/mf0/Connector/R2020b\"],\"version\":\"1.0\"}"
  52X FUEL : Subsystem  VariantControl=52X (FUEL)
      settings: PortSchema="{\"entries\":[{\"content\":{\"headerSize\":26,\"margin\":15,\"minimumSpacing\":25,\"sides\":[{\"content\":{\"connectorIds\":[\"Out7\"]},\"type\":\"ConnectorPlacement.EquallySpacedRectSide\",\"uuid\":\"c62bca68-e99b-4d4a-8c3b-c9a3c6520291\"},{\"content\":{\"connectorIds\":[\"In6\"],\"side\":\"RIGHT\"},\"type\":\"ConnectorPlacement.EquallySpacedRectSide\",\"uuid\":\"9f78cd75-5645-4950-8d66-9f0d33627f1f\"},{\"content\":{\"connectorIds\":[\"Out3\",\"LConn1\",\"Out4\",\"LConn9\",\"LConn2\",\"LConn10\",\"LConn3\",\"Out6\",\"LConn12\",\"LConn6\",\"LConn11\",\"Out1\",\"LConn4\",\"Out2\",\"LConn5\",\"Out5\",\"LConn8\",\"LConn7\",\"In4\",\"LConn13\",\"In2\",\"LConn14\",\"In1\",\"LConn15\",\"LConn16\",\"LConn17\",\"LConn18\",\"In3\",\"LConn19\",\"LConn20\",\"LConn21\",\"In5\",\"LConn22\",\"LConn23\"],\"side\":\"TOP\"},\"type\":\"ConnectorPlacement.EquallySpacedRectSide\",\"uuid\":\"f95077c9-4a6b-4bf1-8b13-59697d659817\"},{\"content\":{\"connectorIds\":[\"RConn1\",\"In7\"],\"side\":\"BOTTOM\"},\"type\":\"ConnectorPlacement.EquallySpacedRectSide\",\"uuid\":\"ebf76d24-9f66-4d93-ad0f-b873a6db50be\"}]},\"type\":\"ConnectorPlacement.EquallySpacedConnector\",\"uuid\":\"da1ef182-4ed3-4fb4-823f-e8eb0a5ecd15\"}],\"packageUris\":[\"http://schema.mathworks.com/mf0/Connector/R2020b\"],\"version\":\"1.0\"}"
  10X-52X : PMIOPort  Side=Right  ConnectionType=Bus: Physical
  522-51XLO : PMIOPort  Port=2  Side=Left  ConnectionType=Bus: LubeOil_P
  523-51XLO : PMIOPort  Port=3  Side=Left  ConnectionType=Bus: LubeOil_P
  524-51XLO : PMIOPort  Port=4  Side=Left  ConnectionType=Bus: LubeOil_P
  523-57XWO : PMIOPort  Port=5  Side=Left  ConnectionType=Bus: WasteOil_P
  20X-525FO : PMIOPort  Port=6  Side=Left  ConnectionType=Bus: FuelOil_P
  30X-526FO : PMIOPort  Port=7  Side=Left  ConnectionType=Bus: FuelOil_P
  50X-522CFW : PMIOPort  Port=8  Side=Left  ConnectionType=Bus: CoolingFW_P
  50X-523CFW : PMIOPort  Port=9  Side=Left  ConnectionType=Bus: CoolingFW_P
  50X-524CFW : PMIOPort  Port=10  Side=Left  ConnectionType=Bus: CoolingFW_P
  50X-528CFW : PMIOPort  Port=11  Side=Left  ConnectionType=Bus: CoolingFW_P
  522-50XCFW : PMIOPort  Port=12  Side=Left  ConnectionType=Bus: CoolingFW_P
  51X-522LO : PMIOPort  Port=13  Side=Left  ConnectionType=Bus: LubeOil_P
  51X-523LO : PMIOPort  Port=14  Side=Left  ConnectionType=Bus: LubeOil_P
  51X-524LO : PMIOPort  Port=15  Side=Left  ConnectionType=Bus: LubeOil_P
  55X-527FO : PMIOPort  Port=16  Side=Left  ConnectionType=Bus: FuelOil_P
  57X-523HP : PMIOPort  Port=17  Side=Left  ConnectionType=Bus: Heat_P
  523-50XCFW : PMIOPort  Port=18  Side=Left  ConnectionType=Bus: CoolingFW_P
  523-57XHP : PMIOPort  Port=19  Side=Left  ConnectionType=Bus: Heat_P
  525-20XFO : PMIOPort  Port=20  Side=Left  ConnectionType=Bus: FuelOil_P
  526-30XFO : PMIOPort  Port=21  Side=Left  ConnectionType=Bus: FuelOil_P
  524-50XCFW : PMIOPort  Port=22  Side=Left  ConnectionType=Bus: CoolingFW_P
  528-50XCFW : PMIOPort  Port=23  Side=Left  ConnectionType=Bus: CoolingFW_P
  527-55XFO : PMIOPort  Port=24  Side=Left  ConnectionType=Bus: FuelOil_P
  52X-20XFO : Outport  OutDataTypeStr=Bus: FuelOil_S
  52X-30XFO : Outport  Port=2  OutDataTypeStr=Bus: FuelOil_S
  52X-50XCFW : Outport  Port=3  OutDataTypeStr=Bus: CoolingFW_S
  52X-51XLO : Outport  Port=4  OutDataTypeStr=Bus: LubeOil_S
  52X-55XFO : Outport  Port=5  OutDataTypeStr=Bus: FuelOil_S
  52X-57XWO : Outport  Port=6  OutDataTypeStr=Bus: WasteOil_S
  528-42XC : Outport  Port=7  OutDataTypeStr=Bus: Control_S

== system SYSTEM/SHIP/500 (AUXILLIARY SYSTEMS)/53X (COMPRESSED AIR) ==
  Bus Element In5 : Inport  PortName=20X-53XCA
  Bus Element In6 : Inport  Port=2  PortName=21X-53XCA
  Bus Element In7 : Inport  Port=3  PortName=22X-53XCA
  Bus Element In8 : Inport  Port=4  PortName=30X-53XCA
  Bus Element In9 : Inport  Port=5  PortName=40X-53XCA
  Bus Element In3 : Inport  Port=6  PortName=50X-53XCFW
  Bus Element In4 : Inport  Port=7  PortName=51X-53XLO
  Bus Element In10 : Inport  Port=8  PortName=54X-53XCA
  Bus Element In11 : Inport  Port=9  PortName=55X-53XCA
  Bus Element In12 : Inport  Port=10  PortName=57X-53XCA
  Bus Element In13 : Inport  Port=11  PortName=59X-53XCA
  Bus Element In2 : Inport  Port=12  PortName=42X-53XC
  Bus Element In1 : Inport  Port=13  PortName=31X-53XP
  10X-53X : PMIOPort  Side=Right  ConnectionType=Bus: Physical
  Bus Element Out4 : Outport  PortName=53X-20XCA
  Bus Element Out5 : Outport  Port=2  PortName=53X-21XCA
  Bus Element Out6 : Outport  Port=3  PortName=53X-22XCA
  Bus Element Out7 : Outport  Port=4  PortName=53X-30XCA
  Bus Element Out8 : Outport  Port=5  PortName=53X-40XCA
  Bus Element Out2 : Outport  Port=6  PortName=53X-50XCFW
  Bus Element Out3 : Outport  Port=7  PortName=53X-51XLO
  Bus Element Out9 : Outport  Port=8  PortName=53X-54XCA
  Bus Element Out10 : Outport  Port=9  PortName=53X-55XCA
  Bus Element Out11 : Outport  Port=10  PortName=53X-57XCA
  Bus Element Out12 : Outport  Port=11  PortName=53X-59XCA
  Bus Element Out1 : Outport  Port=12  PortName=53X-42XC

== system SYSTEM/SHIP/500 (AUXILLIARY SYSTEMS)/54X (BALLAST AND SALTWATER) ==
  Bus Element In5 : Inport  PortName=53X-54XCA
  Bus Element In3 : Inport  Port=2  PortName=50X-54XCFW
  Bus Element In4 : Inport  Port=3  PortName=51X-54XLO
  Bus Element In2 : Inport  Port=4  PortName=42X-54XC
  Bus Element In1 : Inport  Port=5  PortName=31X-54XP
  10X-54X : PMIOPort  Side=Right  ConnectionType=Bus: Physical
  Bus Element Out2 : Outport  PortName=54X-50XSW
  Bus Element Out6 : Outport  Port=2  PortName=54X-51XLO
  Bus Element Out7 : Outport  Port=3  PortName=54X-53XCA
  Bus Element Out3 : Outport  Port=4  PortName=54X-58XSW
  Bus Element Out4 : Outport  Port=5  PortName=54X-57XSW
  Bus Element Out5 : Outport  Port=6  PortName=54X-50XCFW
  Bus Element Out1 : Outport  Port=7  PortName=54X-42XC

== system SYSTEM/SHIP/500 (AUXILLIARY SYSTEMS)/55X (CARGO//MISSION) ==
  Bus Element In3 : Inport  PortName=50X-55XCFW
  Bus Element In4 : Inport  Port=2  PortName=51X-55XLO
  Bus Element In5 : Inport  Port=3  PortName=52X-55XFO
  Bus Element In6 : Inport  Port=4  PortName=53X-55XCA
  Bus Element In2 : Inport  Port=5  PortName=42X-55XC
  Bus Element In1 : Inport  Port=6  PortName=31X-55XP
  10X-55X : PMIOPort  Side=Right  ConnectionType=Bus: Physical
  55X-527FO : PMIOPort  Port=2  Side=Left  ConnectionType=Bus: FuelOil_P
  527-55XFO : PMIOPort  Port=3  Side=Left  ConnectionType=Bus: FuelOil_P
  Bus Element Out2 : Outport  PortName=55X-50XCFW
  Bus Element Out3 : Outport  Port=2  PortName=55X-51XLO
  Bus Element Out4 : Outport  Port=3  PortName=55X-52XFO
  Bus Element Out5 : Outport  Port=4  PortName=55X-53XCA
  Bus Element Out6 : Outport  Port=5  PortName=55X-57XWW
  Bus Element Out7 : Outport  Port=6  PortName=55X-57XWS
  Bus Element Out1 : Outport  Port=7  PortName=55X-42XC

== system SYSTEM/SHIP/500 (AUXILLIARY SYSTEMS)/56X (DECK MACHINERY) ==
  Bus Element In2 : Inport  PortName=42X-56XC
  Bus Element In1 : Inport  Port=2  PortName=31X-56XP
  10X-56X : PMIOPort  Side=Right  ConnectionType=Bus: Physical
  Bus Element Out1 : Outport  PortName=56X-42XC

== system SYSTEM/SHIP/500 (AUXILLIARY SYSTEMS)/57X (WASTE MANAGEMENT) ==
  Bus Element In4 : Inport  PortName=50X-57XCFW
  Bus Element In17 : Inport  Port=2  PortName=20X-57XWG
  Bus Element In18 : Inport  Port=3  PortName=30X-57XWG
  Bus Element In11 : Inport  Port=4  PortName=51X-57XWO
  Bus Element In5 : Inport  Port=5  PortName=51X-57XLO
  Bus Element In12 : Inport  Port=6  PortName=52X-57XWO
  Bus Element In6 : Inport  Port=7  PortName=53X-57XCA
  Bus Element In3 : Inport  Port=8  PortName=54X-57XSW
  Bus Element In10 : Inport  Port=9  PortName=55X-57XWW
  Bus Element In15 : Inport  Port=10  PortName=55X-57XWS
  Bus Element In9 : Inport  Port=11  PortName=59X-57XWW
  Bus Element In16 : Inport  Port=12  PortName=59X-57XWS
  Bus Element In7 : Inport  Port=13  PortName=60X-57XWW
  Bus Element In13 : Inport  Port=14  PortName=60X-57XWS
  Bus Element In8 : Inport  Port=15  PortName=61X-57XWW
  Bus Element In14 : Inport  Port=16  PortName=61X-57XWS
  Bus Element In2 : Inport  Port=17  PortName=42X-57XC
  Bus Element In1 : Inport  Port=18  PortName=31X-57XP
  10X-57X : PMIOPort  Side=Right  ConnectionType=Bus: Physical
  57X-523HP : PMIOPort  Port=2  Side=Left  ConnectionType=Bus: Heat_P
  523-57XHP : PMIOPort  Port=3  Side=Left  ConnectionType=Bus: Heat_P
  523-57XWO : PMIOPort  Port=4  Side=Left  ConnectionType=Bus: WasteOil_P
  Bus Element Out2 : Outport  PortName=57X-50XCFW
  Bus Element Out3 : Outport  Port=2  PortName=57X-51XLO
  Bus Element Out4 : Outport  Port=3  PortName=57X-53XCA
  Bus Element Out1 : Outport  Port=4  PortName=57X-42XC

== system SYSTEM/SHIP/500 (AUXILLIARY SYSTEMS)/58X (FIRE) ==
  Bus Element In4 : Inport  PortName=50X-58XCFW
  Bus Element In5 : Inport  Port=2  PortName=51X-58XLO
  Bus Element In3 : Inport  Port=3  PortName=54X-58XSW
  Bus Element In2 : Inport  Port=4  PortName=42X-58XC
  Bus Element In1 : Inport  Port=5  PortName=31X-58XP
  10X-58X : PMIOPort  Side=Right  ConnectionType=Bus: Physical
  Bus Element Out2 : Outport  PortName=58X-50XCFW
  Bus Element Out3 : Outport  Port=2  PortName=58X-51XLO
  Bus Element Out1 : Outport  Port=3  PortName=58X-42XC

== system SYSTEM/SHIP/500 (AUXILLIARY SYSTEMS)/59X (HOTEL) ==
  Bus Element In5 : Inport  PortName=50X-59XCFW
  Bus Element In6 : Inport  Port=2  PortName=51X-59XLO
  Bus Element In7 : Inport  Port=3  PortName=53X-59XCA
  Bus Element In2 : Inport  Port=4  PortName=42X-59XC
  Bus Element In3 : Inport  Port=5  PortName=60X-59XC
  Bus Element In4 : Inport  Port=6  PortName=61X-59XC
  Bus Element In1 : Inport  Port=7  PortName=31X-59XP
  10X-59X : PMIOPort  Side=Right  ConnectionType=Bus: Physical
  Bus Element Out4 : Outport  PortName=59X-50XCFW
  Bus Element Out5 : Outport  Port=2  PortName=59X-51XLO
  Bus Element Out6 : Outport  Port=3  PortName=59X-53XCA
  Bus Element Out7 : Outport  Port=4  PortName=59X-57XWW
  Bus Element Out8 : Outport  Port=5  PortName=59X-57XWS
  Bus Element Out1 : Outport  Port=6  PortName=59X-42XC
  Bus Element Out2 : Outport  Port=7  PortName=59X-60XC
  Bus Element Out3 : Outport  Port=8  PortName=59X-61XC

== system SYSTEM/SHIP/600 (OUTFITTING)/60X (ACCOMODATION) ==
  Bus Element In3 : Inport  PortName=50X-60XCFW
  Bus Element In2 : Inport  Port=2  PortName=59X-60XC
  Bus Element In1 : Inport  Port=3  PortName=31X-60XP
  10X-60X : PMIOPort  Side=Right  ConnectionType=Bus: Physical
  Bus Element Out2 : Outport  PortName=60X-50XCFW
  Bus Element Out3 : Outport  Port=2  PortName=60X-57XWW
  Bus Element Out4 : Outport  Port=3  PortName=60X-57XWS
  Bus Element Out1 : Outport  Port=4  PortName=60X-59XC

== system SYSTEM/SHIP/600 (OUTFITTING)/61X (SHOPS) ==
  Bus Element In3 : Inport  PortName=50X-61XCFW
  Bus Element In2 : Inport  Port=2  PortName=59X-61XC
  Bus Element In1 : Inport  Port=3  PortName=31X-61XP
  10X-61X : PMIOPort  Side=Right  ConnectionType=Bus: Physical
  Bus Element Out2 : Outport  PortName=61X-50XCFW
  Bus Element Out3 : Outport  Port=2  PortName=61X-57XWW
  Bus Element Out4 : Outport  Port=3  PortName=61X-57XWS
  Bus Element Out1 : Outport  Port=4  PortName=61X-59XC

== system SYSTEM/SHIP/600 (OUTFITTING)/62X (LSA) ==
  10X-62X : PMIOPort  Side=Right  ConnectionType=Bus: Physical

== system SYSTEM/SHIP/700 (WEAPONS)/70X (ASW) ==
  Bus Element In2 : Inport  PortName=42X-70XC
  Bus Element In1 : Inport  Port=2  PortName=31X-70XP
  10X-70X : PMIOPort  Side=Right  ConnectionType=Bus: Physical
  Bus Element Out1 : Outport  PortName=70X-42XC

== system SYSTEM/SHIP/700 (WEAPONS)/71X (SS) ==
  Bus Element In3 : Inport  PortName=50X-71XCFW
  Bus Element In2 : Inport  Port=2  PortName=42X-71XC
  Bus Element In1 : Inport  Port=3  PortName=31X-71XP
  10X-71X : PMIOPort  Side=Right  ConnectionType=Bus: Physical
  Bus Element Out2 : Outport  PortName=71X-50XCFW
  Bus Element Out1 : Outport  Port=2  PortName=71X-42XC

== system SYSTEM/SHIP/700 (WEAPONS)/72X (SA) ==
  Bus Element In3 : Inport  PortName=50X-72XCFW
  Bus Element In2 : Inport  Port=2  PortName=42X-72XC
  Bus Element In1 : Inport  Port=3  PortName=31X-72XP
  10X-72X : PMIOPort  Side=Right  ConnectionType=Bus: Physical
  Bus Element Out2 : Outport  PortName=72X-50XCFW
  Bus Element Out1 : Outport  Port=2  PortName=72X-42XC

== system SYSTEM/SHIP/700 (WEAPONS)/73X (EW) ==
  Bus Element In3 : Inport  PortName=50X-73XCFW
  Bus Element In2 : Inport  Port=2  PortName=42X-73XC
  Bus Element In1 : Inport  Port=3  PortName=31X-73XP
  10X-73X : PMIOPort  Side=Right  ConnectionType=Bus: Physical
  Bus Element Out2 : Outport  PortName=73X-50XCFW
  Bus Element Out1 : Outport  Port=2  PortName=73X-42XC

== system SYSTEM/SHIP/700 (WEAPONS)/74X (COUNTERMEASURES) ==
  Bus Element In2 : Inport  PortName=42X-74XC
  Bus Element In1 : Inport  Port=2  PortName=31X-74XP
  10X-74X : PMIOPort  Side=Right  ConnectionType=Bus: Physical
  Bus Element Out1 : Outport  PortName=74X-42XC

== system SYSTEM/SHIP/200 (PROPULSION)/20X (MAIN ENGINE)/20X ABSENT ==

== system SYSTEM/SHIP/200 (PROPULSION)/20X (MAIN ENGINE)/20X DIESEL ENGINE ==
  Bus Element In1 : Inport  PortName=42X-20XC
  Bus Element In3 : Inport  Port=2  PortName=51X-20XLO
  Bus Element In4 : Inport  Port=3  PortName=52X-20XFO
  Bus Element In5 : Inport  Port=4  PortName=53X-20XCA
  Bus Element In2 : Inport  Port=5  PortName=50X-20XCFW
  20X-525FO : PMIOPort  Side=Left  ConnectionType=Bus: FuelOil_P
  525-20XFO : PMIOPort  Port=2  Side=Left  ConnectionType=Bus: FuelOil_P
  TO 23X : PMIOPort  Port=3  Side=Left  ConnectionType=Bus: Physical
  10X-20X : PMIOPort  Port=4  Side=Right  ConnectionType=Bus: Physical
  FROM 20X : PMIOPort  Port=5  Side=Right  ConnectionType=Bus: Physical
  Bus Element Out1 : Outport  PortName=20X-42XC
  Bus Element Out3 : Outport  Port=2  PortName=20X-51XLO
  Bus Element Out4 : Outport  Port=3  PortName=20X-52XFO
  Bus Element Out5 : Outport  Port=4  PortName=20X-53XCA
  Bus Element Out6 : Outport  Port=5  PortName=20X-57XWG
  Bus Element Out2 : Outport  Port=6  PortName=20X-50XCFW

== system SYSTEM/SHIP/200 (PROPULSION)/21X (PROPULSORS)/21X ABSENT ==

== system SYSTEM/SHIP/200 (PROPULSION)/21X (PROPULSORS)/21X ELECTRIC DRIVE ==
  Bus Element In1 : Inport  PortName=42X-21XC
  Bus Element In3 : Inport  Port=2  PortName=51X-21XLO
  Bus Element In4 : Inport  Port=3  PortName=53X-21XCA
  Bus Element In2 : Inport  Port=4  PortName=50X-21XCFW
  10X-21X : PMIOPort  Side=Right  ConnectionType=Bus: Physical
  FROM 22X : PMIOPort  Port=2  Side=Right  ConnectionType=Bus: Physical
  Bus Element Out1 : Outport  PortName=21X-42XC
  Bus Element Out3 : Outport  Port=2  PortName=21X-51XLO
  Bus Element Out4 : Outport  Port=3  PortName=21X-53XCA
  Bus Element Out2 : Outport  Port=4  PortName=21X-50XCFW

== system SYSTEM/SHIP/200 (PROPULSION)/21X (PROPULSORS)/21X ELECTRIC DRIVE + MANEUVERING THRUSTER ==
  Bus Element In1 : Inport  PortName=42X-21XC
  Bus Element In3 : Inport  Port=2  PortName=51X-21XLO
  Bus Element In4 : Inport  Port=3  PortName=53X-21XCA
  Bus Element In2 : Inport  Port=4  PortName=50X-21XCFW
  10X-21X : PMIOPort  Side=Right  ConnectionType=Bus: Physical
  FROM 22X : PMIOPort  Port=2  Side=Right  ConnectionType=Bus: Physical
  Bus Element Out1 : Outport  PortName=21X-42XC
  Bus Element Out3 : Outport  Port=2  PortName=21X-51XLO
  Bus Element Out4 : Outport  Port=3  PortName=21X-53XCA
  Bus Element Out2 : Outport  Port=4  PortName=21X-50XCFW

== system SYSTEM/SHIP/200 (PROPULSION)/21X (PROPULSORS)/21X SHAFT DRIVE ==
  Bus Element In1 : Inport  PortName=42X-21XC
  Bus Element In3 : Inport  Port=2  PortName=51X-21XLO
  Bus Element In4 : Inport  Port=3  PortName=53X-21XCA
  Bus Element In2 : Inport  Port=4  PortName=50X-21XCFW
  10X-21X : PMIOPort  Side=Right  ConnectionType=Bus: Physical
  FROM 22X : PMIOPort  Port=2  Side=Right  ConnectionType=Bus: Physical
  Bus Element Out1 : Outport  PortName=21X-42XC
  Bus Element Out3 : Outport  Port=2  PortName=21X-51XLO
  Bus Element Out4 : Outport  Port=3  PortName=21X-53XCA
  Bus Element Out2 : Outport  Port=4  PortName=21X-50XCFW

== system SYSTEM/SHIP/200 (PROPULSION)/21X (PROPULSORS)/21X SHAFT DRIVE + MANEUVERING THRUSTER ==
  Bus Element In1 : Inport  PortName=42X-21XC
  Bus Element In3 : Inport  Port=2  PortName=51X-21XLO
  Bus Element In4 : Inport  Port=3  PortName=53X-21XCA
  Bus Element In2 : Inport  Port=4  PortName=50X-21XCFW
  10X-21X : PMIOPort  Side=Right  ConnectionType=Bus: Physical
  FROM 22X : PMIOPort  Port=2  Side=Right  ConnectionType=Bus: Physical
  Bus Element Out1 : Outport  PortName=21X-42XC
  Bus Element Out3 : Outport  Port=2  PortName=21X-51XLO
  Bus Element Out4 : Outport  Port=3  PortName=21X-53XCA
  Bus Element Out2 : Outport  Port=4  PortName=21X-50XCFW

== system SYSTEM/SHIP/200 (PROPULSION)/21X (PROPULSORS)/21X WATER JET ==
  Bus Element In1 : Inport  PortName=42X-21XC
  Bus Element In3 : Inport  Port=2  PortName=51X-21XLO
  Bus Element In4 : Inport  Port=3  PortName=53X-21XCA
  Bus Element In2 : Inport  Port=4  PortName=50X-21XCFW
  10X-21X : PMIOPort  Side=Right  ConnectionType=Bus: Physical
  FROM 22X : PMIOPort  Port=2  Side=Right  ConnectionType=Bus: Physical
  Bus Element Out1 : Outport  PortName=21X-42XC
  Bus Element Out3 : Outport  Port=2  PortName=21X-51XLO
  Bus Element Out4 : Outport  Port=3  PortName=21X-53XCA
  Bus Element Out2 : Outport  Port=4  PortName=21X-50XCFW
